simulink model "first_order_system_step"  (R2022b)
settings: Solver=VariableStepAuto  StartTime=0.0  StopTime=10  MaxStep=1e-3  RelTol=1e-3
settings Model: Creator=yasso  LastModifiedBy=yasso

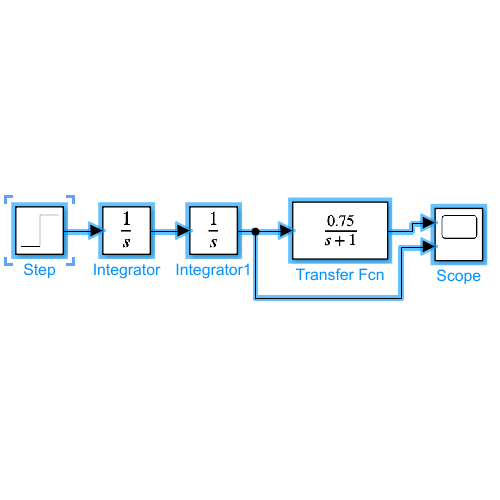
[thumbnail: Simulink's stored preview of the top-level diagram]
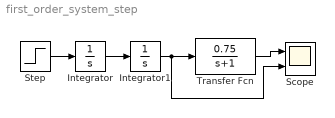
== system first_order_system_step ==
  Integrator : Integrator
  Integrator1 : Integrator
  Scope : Scope  NumInputPorts=2
  Step : Step  SampleTime=0
  Transfer Fcn : TransferFcn  Numerator=[0 0.75]  Denominator=[1 1]
  wires:
  Step/1 -> Integrator/1
  Transfer Fcn/1 -> Scope/1
  Integrator/1 -> Integrator1/1
  Integrator1/1 -> Scope/2, Transfer Fcn/1
